simulink model "Simple_Algorithm"  (R2012b)
settings: Solver=ode45  StartTime=0.0  StopTime=10.0  RelTol=1e-3
settings Model: Creator=Ahmad  LastModifiedBy=Ahmad

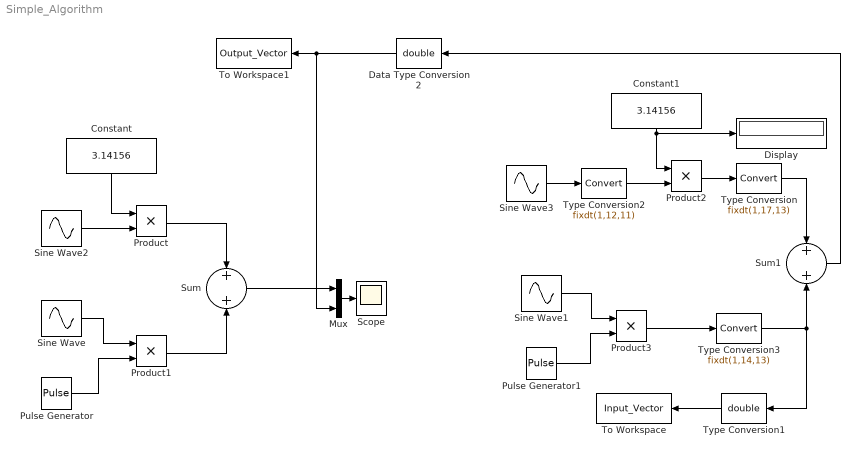
== system Simple_Algorithm ==
  Constant : Constant  Value=3.14156  VectorParams1D=off  OutDataTypeStr=double  SampleTime=1/100e6
  Constant1 : Constant  Value=3.14156  OutDataTypeStr=fixdt(1,9,6)  SampleTime=1/100e6
  Data Type Conversion2 : DataTypeConversion  OutDataTypeStr=double
  Display : Display
  Mux : Mux  Inputs=2
  Product{,1..3} (4 alike) : Product  RndMeth=Zero
  Pulse Generator : DiscretePulseGenerator  Period=100  PulseWidth=50  SampleTime=1/100e6
  Pulse Generator1 : DiscretePulseGenerator  Period=100  PulseWidth=50  SampleTime=1/100e6
  Scope : Scope
      settings: TimeRange=7.000000000000062e-05  YMin=-3  YMax=4
  Sine Wave : Sin  Amplitude=0.9  Frequency=2*pi*1e6  SampleTime=1/100e6
  Sine Wave1 : Sin  Amplitude=0.9  Frequency=2*pi*1e6  SampleTime=1/100e6
  Sine Wave2 : Sin  Frequency=2*pi*2e6  SampleTime=1/100e6
  Sine Wave3 : Sin  Frequency=2*pi*2e6  SampleTime=1/100e6
  Sum : Sum  Inputs=+|+
  Sum1 : Sum  Inputs=+|+
  To Workspace : ToWorkspace  VariableName=Input_Vector  SampleTime=-1  SaveFormat=Timeseries
  To Workspace1 : ToWorkspace  VariableName=Output_Vector  SampleTime=-1  SaveFormat=Timeseries
  Type Conversion : DataTypeConversion  OutDataTypeStr=fixdt(1,17,13)
  Type Conversion1 : DataTypeConversion  OutDataTypeStr=double
  Type Conversion2 : DataTypeConversion  OutDataTypeStr=fixdt(1,12,11)
  Type Conversion3 : DataTypeConversion  OutDataTypeStr=fixdt(1,14,13)
  wires:
  Constant/1 -> Product/1
  Sine Wave2/1 -> Product/2
  Product/1 -> Sum/1
  Sine Wave/1 -> Product1/1
  Pulse Generator/1 -> Product1/2
  Constant1/1 -> Product2/1, Display/1
  Type Conversion2/1 -> Product2/2
  Product2/1 -> Type Conversion/1
  Sum1/1 -> Data Type Conversion2/1
  Type Conversion/1 -> Sum1/1
  Mux/1 -> Scope/1
  Sum/1 -> Mux/1
  Data Type Conversion2/1 -> To Workspace1/1, Mux/2
  Product1/1 -> Sum/2
  Type Conversion3/1 -> Sum1/2, Type Conversion1/1
  Product3/1 -> Type Conversion3/1
  Sine Wave1/1 -> Product3/1
  Pulse Generator1/1 -> Product3/2
  Sine Wave3/1 -> Type Conversion2/1
  Type Conversion1/1 -> To Workspace/1
